simulink model "test_bench"  (R2021b)
settings: Solver=FixedStepAuto  StartTime=0.0  StopTime=10  FixedStep=Ts  RelTol=1e-3
libraries: cstblocks x1, simulink x1
settings Model: Creator=antony  LastModifiedBy=antony

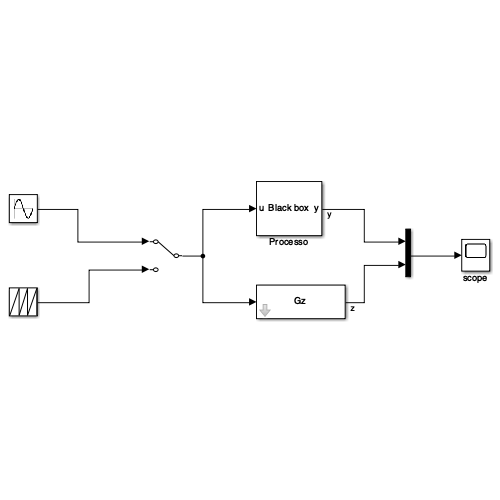
[thumbnail: Simulink's stored preview of the top-level diagram]
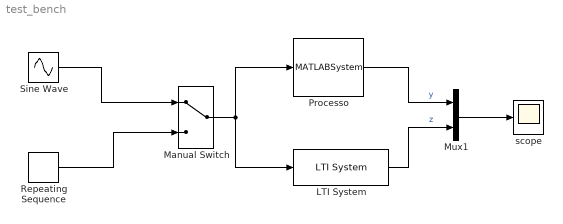
== system test_bench ==
  LTI System : cstblocks/LTI System  sys=Gz  IC=[]
  Manual Switch : ManualSwitch
  Mux1 : Mux  Inputs=2
  Processo : MATLABSystem  System=linSysObj  SimulateUsing=Interpreted execution
      mask Type: linSysObj
      mask Display:
      | disp('Black box');
      | port_label('input',1,'u');
      | port_label('output',1,'y');
  Repeating Sequence : simulink/Sources/Repeating Sequence  rep_seq_t=[0 1]  rep_seq_y=[-5 5]
  Sine Wave : Sin  Phase=pi  SampleTime=0
  scope : Scope
  wires:
  Processo/1 -> Mux1/1  "y"
  Manual Switch/1 -> LTI System/1, Processo/1
  LTI System/1 -> Mux1/2  "z"
  Repeating Sequence/1 -> Manual Switch/2
  Mux1/1 -> scope/1
  Sine Wave/1 -> Manual Switch/1
